simulink model "luu_tam"  (R2019a)
settings: Solver=VariableStepAuto  StartTime=0.0  StopTime=10.0  RelTol=1e-3
undefined symbols (not defined in the file): K
settings Model: Creator=chute  LastModifiedBy=chute

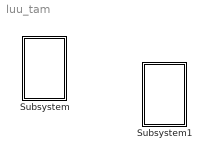
== system luu_tam ==
  Subsystem : Subsystem
  Subsystem1 : Subsystem

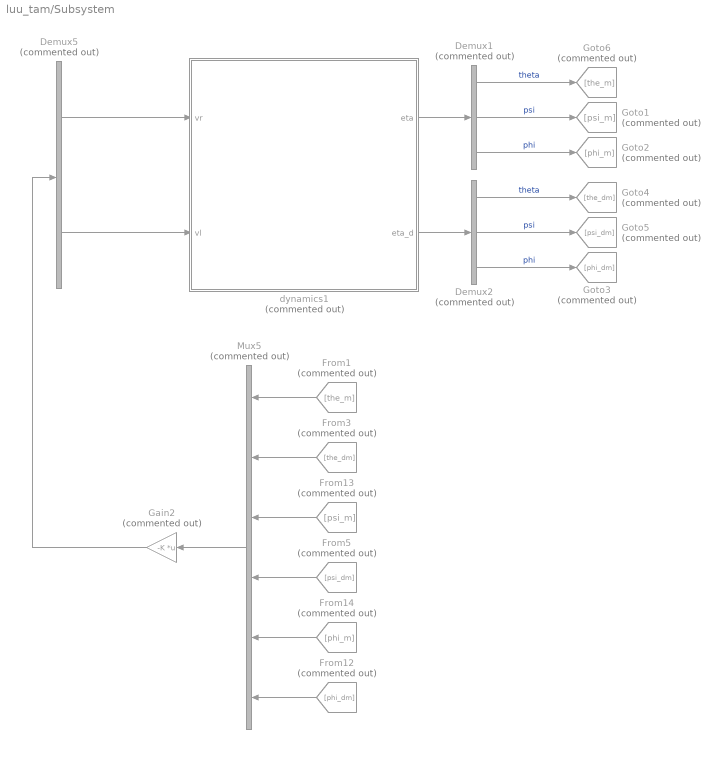
== system luu_tam/Subsystem ==
  Demux1 : Demux  Commented=on  Outputs=3
  Demux2 : Demux  Commented=on  Outputs=3
  Demux5 : Demux  Commented=on  Outputs=2
  From1 : From  Commented=on  GotoTag=the_m
  From12 : From  Commented=on  GotoTag=phi_dm
  From13 : From  Commented=on  GotoTag=psi_m
  From14 : From  Commented=on  GotoTag=phi_m
  From3 : From  Commented=on  GotoTag=the_dm
  From5 : From  Commented=on  GotoTag=psi_dm
  Gain2 : Gain  Commented=on  Gain=-K  Multiplication=Matrix(K*u) (u vector)
  Goto1 : Goto  Commented=on  GotoTag=psi_m
  Goto2 : Goto  Commented=on  GotoTag=phi_m
  Goto3 : Goto  Commented=on  GotoTag=phi_dm
  Goto4 : Goto  Commented=on  GotoTag=the_dm
  Goto5 : Goto  Commented=on  GotoTag=psi_dm
  Goto6 : Goto  Commented=on  GotoTag=the_m
  Mux5 : Mux  Commented=on  Inputs=6
  dynamics1 : Subsystem  Commented=on
  wires:
  From12/1 -> Mux5/6
  Demux1/2 -> Goto1/1  "psi"
  Demux2/1 -> Goto4/1  "theta"
  dynamics1/2(eta_d) -> Demux2/1
  Demux2/2 -> Goto5/1  "psi"
  From1/1 -> Mux5/1
  Mux5/1 -> Gain2/1
  From3/1 -> Mux5/2
  Gain2/1 -> Demux5/1
  Demux5/2 -> dynamics1/2(vl)
  Demux2/3 -> Goto3/1  "phi"
  Demux5/1 -> dynamics1/1(vr)
  From5/1 -> Mux5/4
  From14/1 -> Mux5/5
  From13/1 -> Mux5/3
  Demux1/1 -> Goto6/1  "theta"
  dynamics1/1(eta) -> Demux1/1
  Demux1/3 -> Goto2/1  "phi"

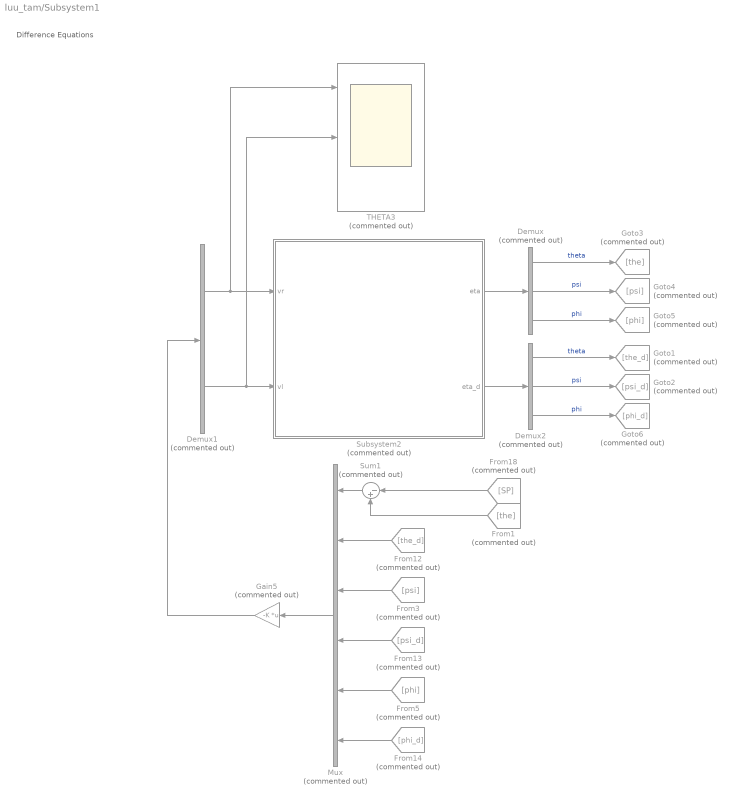
== system luu_tam/Subsystem1 ==
  note: Difference Equations
  Demux : Demux  Commented=on  Outputs=3
  Demux1 : Demux  Commented=on  Outputs=2
  Demux2 : Demux  Commented=on  Outputs=3
  From1 : From  Commented=on  GotoTag=the
  From12 : From  Commented=on  GotoTag=the_d
  From13 : From  Commented=on  GotoTag=psi_d
  From14 : From  Commented=on  GotoTag=phi_d
  From18 : From  Commented=on  GotoTag=SP
  From3 : From  Commented=on  GotoTag=psi
  From5 : From  Commented=on  GotoTag=phi
  Gain5 : Gain  Commented=on  Gain=-K  Multiplication=Matrix(K*u) (u vector)
  Goto1 : Goto  Commented=on  GotoTag=the_d
  Goto2 : Goto  Commented=on  GotoTag=psi_d
  Goto3 : Goto  Commented=on  GotoTag=the
  Goto4 : Goto  Commented=on  GotoTag=psi
  Goto5 : Goto  Commented=on  GotoTag=phi
  Goto6 : Goto  Commented=on  GotoTag=phi_d
  Mux : Mux  Commented=on  Inputs=6
  Subsystem2 : Subsystem  Commented=on
  Sum1 : Sum  Commented=on  Inputs=|-+
  THETA3 : Scope  Commented=on  NumInputPorts=3
  wires:
  Demux2/3 -> Goto6/1  "phi"
  Demux2/1 -> Goto1/1  "theta"
  Gain5/1 -> Demux1/1
  Mux/1 -> Gain5/1
  Demux1/1 -> THETA3/1, Subsystem2/1(vr)
  Subsystem2/1(eta) -> Demux/1
  From18/1 -> Sum1/1
  From3/1 -> Mux/3
  From12/1 -> Mux/2
  Demux/1 -> Goto3/1  "theta"
  From14/1 -> Mux/6
  Demux/3 -> Goto5/1  "phi"
  Demux1/2 -> THETA3/2, Subsystem2/2(vl)
  Demux2/2 -> Goto2/1  "psi"
  Demux/2 -> Goto4/1  "psi"
  From5/1 -> Mux/5
  Subsystem2/2(eta_d) -> Demux2/1
  From1/1 -> Sum1/2
  Sum1/1 -> Mux/1
  From13/1 -> Mux/4

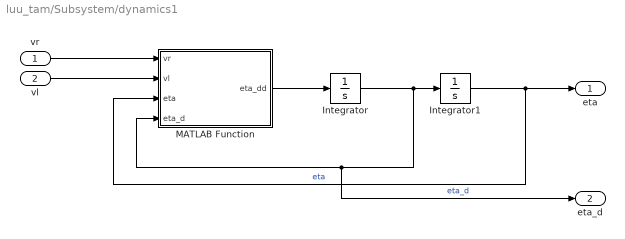
== system luu_tam/Subsystem/dynamics1 ==
  vr : Inport
  vl : Inport  Port=2
  Integrator : Integrator  InitialCondition=[0.01;0.01;0]
  Integrator1 : Integrator  InitialCondition=[0.01;0.01;0]
  MATLAB Function : MATLAB Function  TreatAsAtomicUnit=on
  eta : Outport
  eta_d : Outport  Port=2
  wires:
  Integrator/1 -> Integrator1/1, eta_d/1, MATLAB Function/4(eta_d)  "eta_d"
  Integrator1/1 -> eta/1, MATLAB Function/3(eta)  "eta"
  MATLAB Function/1(eta_dd) -> Integrator/1
  vr/1 -> MATLAB Function/1(vr)
  vl/1 -> MATLAB Function/2(vl)

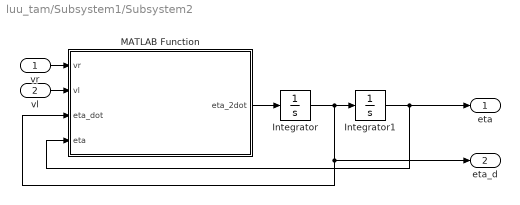
== system luu_tam/Subsystem1/Subsystem2 ==
  vr : Inport
  vl : Inport  Port=2
  Integrator : Integrator  InitialCondition=[0.01;0.01;0]
  Integrator1 : Integrator  InitialCondition=[0.01;0.01;0]
  MATLAB Function : MATLAB Function  TreatAsAtomicUnit=on
  eta : Outport
  eta_d : Outport  Port=2
  wires:
  vl/1 -> MATLAB Function/2(vl)
  MATLAB Function/1(eta_2dot) -> Integrator/1
  Integrator/1 -> eta_d/1, MATLAB Function/3(eta_dot), Integrator1/1
  Integrator1/1 -> eta/1, MATLAB Function/4(eta)
  vr/1 -> MATLAB Function/1(vr)

== matlab function luu_tam/Subsystem/dynamics1/MATLAB Function ==
  data: vr input; vl input; eta_dd output; eta input; eta_d input
function eta_dd= fcn(vr,vl,eta,eta_d)
%% declare the parameter:
% g =9.81; % gravity acceleration
% m =0.046; % wheel weight
% R =0.3375; % Wheel radius
% M =0.95;  % body weight
% W =0.22; % Body width
% D =0.1; % Body depth
% H =0.121;% Body Height
% L =0.121/2;% distance
% 
% J_psi  = M*L^2/3; % Body inertia moment
% Jw = m*R^2/2;  %Wheel inertia moment
% J_phi = M*(W^2+D^2)/12; % Body yaw inertia moment
% Jm = 0.041185; % Dc motor inertia moment
% 
% n =30 ; %gear ratio



%% Ning

% anp = (n*Kt)/Rm;
% bet = (n*Kt*Kb)/Rm+fm;
% 
% x1=0;x2=0;x3=0;x6=0;x9=0;x4=0;x5=0;x7=0;x8=0;
% m= 0.04; n=20; R=0.0325;M=0.8;L=0.0628; Jw = m*R^2/2; J_psi = M*L^2/3;
% Rm = 1.5628; Kt = 0.023385; Jm = 1.175e-05; Kb = 5.9233e-07; anp = n*Kt/Rm; fm=0.0022;
% bet = n*Kt*Kb/Rm + fm;
% W = 0.168;
% fw = 0.0000001;
% D = 0.098;
% J_phi = M*(W^2+D^2)/12;
% g = 9.81;


%% Hoang

g =9.81; % gravity acceleration
m =0.046; % wheel weight
R =0.0335; % Wheel radius
M =0.945;  % body weight
W =0.17; % Body width
D =0.1; % Body depth
H =0.121;% Body Height
L =0.121/2;% distance

J_psi  = M*L^2/3; % Body inertia moment
Jw = m*R^2/2;  %Wheel inertia moment
J_phi = M*(W^2+D^2)/12; % Body yaw inertia moment
Jm = 0.041185; % Dc motor inertia moment

n =30 ; %gear ratio
Rm=8.6123;      %dien tro dong co DC
Kb=0.22244;   %he so emf cua dong co
Kt=3.0896;   %momemt xoan cua dong co DC\
fm = 0.0022; % friction cof between body and DC motor.
fw = 0; % friction cof between wheel and floor
anp = (n*Kt)/Rm;
bet = (n*Kt*Kb/Rm)+fm;

%notation:
the=eta(1,1);
psi=eta(2,1);
phi=eta(3,1);

the_dot=eta_d(1,1);
psi_dot=eta_d(2,1);
phi_dot=eta_d(3,1);





%% DC Motor
F_the = anp*(vl+vr)-2*(bet+fw)*the_dot+2*bet*psi_dot;
F_psi = -anp*(vl+vr)+2*bet*the_dot-2*bet*psi_dot;
F_phi = W*anp*(vr-vl)/(2*R)-W^2*((bet+fw)*phi_dot)/2*R^2;
tor =[F_the;F_psi;F_phi];
%% dyn
% Mass matrix:
M1 = ...
[2*Jw + 2*Jm*n^2 + R^2*(M + 2*m),L*M*R*cos(psi) - 2*Jm*n^2,0;
 L*M*R*cos(psi) - 2*Jm*n^2,J_psi + L^2*M + 2*Jm*n^2,0;
 0,0,J_phi + (W^2*m)/2 + L^2*M*sin(psi)^2 + (W^2*(Jw + Jm*n^2))/(2*R^2)];

%Coriolis matrix:
C1 = ...
[0,-L*M*R*psi_dot*sin(psi),0;
 0,0,-(L^2*M*phi_dot*sin(2*psi))/2;
 0,(L^2*M*phi_dot*sin(2*psi))/2,(L^2*M*psi_dot*sin(2*psi))/2];




% Gravity vector:
G1=...
[0;
-L*M*g*sin(psi);
0];

% Fv: viscous friction 2
% Fc: Coulomb friction 2
Fv=0.01*diag([1,1,1]);
Fc = 0.01*diag([1,1,1]);
dt = Fc*sign(eta_d) + Fv*eta_d;
eta_dd=inv(M1)*(tor-C1*eta_d-G1);


end

== matlab function luu_tam/Subsystem1/Subsystem2/MATLAB Function ==
  data: vr input; eta_2dot output; vl input; eta_dot input; eta input
function eta_2dot  = fcn(vr,vl,eta_dot,eta)
%% Declare the parameter:
%% Hoang

g =9.81; % gravity acceleration
m =0.046; % wheel weight
R =0.0335; % Wheel radius
M =0.945;  % body weight
W =0.17; % Body width
D =0.1; % Body depth
H =0.121;% Body Height
L =0.121/2;% distance

J_psi  = M*L^2/3; % Body inertia moment
Jw = m*R^2/2;  %Wheel inertia moment
J_phi = M*(W^2+D^2)/12; % Body yaw inertia moment
Jm = 0.041185; % Dc motor inertia moment

n =30 ; %gear ratio
Rm=8.6123;      %dien tro dong co DC
Kb=0.22244;   %he so emf cua dong co
Kt=3.0896;   %momemt xoan cua dong co DC\
fm = 0.0022; % friction cof between body and DC motor.
fw = 0; % friction cof between wheel and floor
anp = (n*Kt)/Rm;
bet = (n*Kt*Kb/Rm)+fm;
%% notation:
the_dot=eta_dot(1,1);
psi_dot=eta_dot(2,1);
phi_dot=eta_dot(3,1);

the=eta(1,1);
psi=eta(2,1);
phi=eta(3,1);



the_2dot = (J_psi*anp*vl + J_psi*anp*vr - 2*J_psi*bet*the_dot + 2*J_psi*bet*psi_dot - 2*J_psi*fw*the_dot + L^2*M*anp*vl + L^2*M*anp*vr - 2*L^2*M*bet*the_dot + 2*L^2*M*bet*psi_dot - 2*L^2*M*fw*the_dot - 4*Jm*fw*n^2*the_dot + L^3*M^2*R*psi_dot^2*sin(psi) - 2*L*M*R*bet*the_dot*cos(psi) + 2*L*M*R*bet*psi_dot*cos(psi) - L^3*M^2*R*phi_dot^2*sin(2*psi)*cos(psi) - L^2*M^2*R*g*cos(psi)*sin(psi) + J_psi*L*M*R*psi_dot^2*sin(psi) + 2*Jm*L*M*g*n^2*sin(psi) + 2*Jm*L^2*M*n^2*phi_dot^2*sin(2*psi) + L*M*R*anp*vl*cos(psi) + L*M*R*anp*vr*cos(psi) + 2*Jm*L*M*R*n^2*psi_dot^2*sin(psi))/(2*J_psi*Jw + L^2*M^2*R^2 + 2*Jw*L^2*M + J_psi*M*R^2 + 2*J_psi*Jm*n^2 + 4*Jm*Jw*n^2 + 2*J_psi*R^2*m + 2*Jm*L^2*M*n^2 + 2*Jm*M*R^2*n^2 + 2*L^2*M*R^2*m + 4*Jm*R^2*m*n^2 - L^2*M^2*R^2*cos(psi)^2 + 4*Jm*L*M*R*n^2*cos(psi));
psi_2dot =-(2*Jw*anp*vl + 2*Jw*anp*vr - 4*Jw*bet*the_dot + 4*Jw*bet*psi_dot + M*R^2*anp*vl + M*R^2*anp*vr - 2*M*R^2*bet*the_dot + 2*M*R^2*bet*psi_dot + 2*R^2*anp*m*vl + 2*R^2*anp*m*vr + 4*Jm*fw*n^2*the_dot - 4*R^2*bet*m*the_dot + 4*R^2*bet*m*psi_dot - L*M^2*R^2*g*sin(psi) - 2*Jw*L*M*g*sin(psi) - 2*L*M*R*bet*the_dot*cos(psi) + 2*L*M*R*bet*psi_dot*cos(psi) - 2*L*M*R*fw*the_dot*cos(psi) + L^2*M^2*R^2*psi_dot^2*cos(psi)*sin(psi) - L^2*M^2*R^2*phi_dot^2*cos(psi)*sin(psi) - 2*Jw*L^2*M*phi_dot^2*cos(psi)*sin(psi) - 2*Jm*L*M*g*n^2*sin(psi) - 2*L*M*R^2*g*m*sin(psi) + L*M*R*anp*vl*cos(psi) + L*M*R*anp*vr*cos(psi) - 2*Jm*L^2*M*n^2*phi_dot^2*cos(psi)*sin(psi) - 2*L^2*M*R^2*m*phi_dot^2*cos(psi)*sin(psi) - 2*Jm*L*M*R*n^2*psi_dot^2*sin(psi))/(2*J_psi*Jw + L^2*M^2*R^2 + 2*Jw*L^2*M + J_psi*M*R^2 + 2*J_psi*Jm*n^2 + 4*Jm*Jw*n^2 + 2*J_psi*R^2*m + 2*Jm*L^2*M*n^2 + 2*Jm*M*R^2*n^2 + 2*L^2*M*R^2*m + 4*Jm*R^2*m*n^2 - L^2*M^2*R^2*cos(psi)^2 + 4*Jm*L*M*R*n^2*cos(psi));
phi_2dot = -(W^2*bet*phi_dot + W^2*fw*phi_dot + R*W*anp*vl - R*W*anp*vr + 4*L^2*M*R^2*psi_dot*phi_dot*cos(psi)*sin(psi))/(2*J_phi*R^2 + Jw*W^2 + Jm*W^2*n^2 + R^2*W^2*m + 2*L^2*M*R^2*sin(psi)^2);
eta_2dot=[the_2dot;psi_2dot;phi_2dot];
end
